simulink model "sdruqpskrx"  (R2025b)
settings: Solver=FixedStepDiscrete  StartTime=0.0  StopTime=inf  RelTol=1e-3
PreLoadFcn:
  | platform = sdruExampleFindRadio;
  | sdrqpskrx = sdruQPSKReceiverSLInit(platform, false, true);
  | clear platform
PostLoadFcn:
  | sdruExampleSetAvailableRadio;
InitFcn:
  | platform = get_param([gcs '/USRP Receiver'], 'Platform');
  | sdrqpskrx = sdruQPSKReceiverSLInit(platform, false, true);
  | switch platform
  |   case 'X300'
  |     set_param([gcs,'/USRP Receiver'], 'masterClkRateX300','200e6');
  |   case 'X310'
  |     set_param([gcs,'/USRP Receiver'], 'masterClkRateX310','200e6');
  |   case 'X410'
  |     set_param([gcs,'/USRP Receiver'], 'masterClkRateX410','250e6');
  |   case 'E320'
  |     set_param([gcs,'/USRP Receiver'], 'masterClkRateE320','50e6');
  |   case 'N300'
  |     set_param([gcs,'/USRP Receiver'], 'masterClkRateN300','125e6');
  |   case 'N310'
  |     set_param([gcs,'/USRP Receiver'], 'masterClkRateN310','125e6');
  |   case 'N320/N321'
  |      set_param([gcs,'/USRP Receiver'], 'masterClkRateN320','200e6');
  | end
  | clear platform
undefined symbols (not defined in the file): RX, TX
libraries: commrfcorlib x2, dspstat3 x2, commdigbbndpm3 x2, commsync2 x2, commrflib2 x1, dspsigops x1, simulink x1, commsequence2 x1, commsink2 x1, commutil2 x1, dspsrcs4 x1, commfilt2 x1
settings Model: FPTRunName=Active  SimulationMode=accelerator  Creator=The MathWorks, Inc.  LastModifiedBy=MiguelG
settings SolverCC: AlgebraicLoopSolver=TrustRegion  AutoInsertRateTranBlk=on  MaxZcPerStep=1.0
settings DataIOCC: LimitDataPoints=on  SaveFormat=Structure  SaveOutput=off  SignalLogging=off  DSMLogging=off  SaveTime=off  ReturnWorkspaceOutputs=off
settings OptimizationCC: DefaultParameterBehavior=Inlined  ReuseModelBlockBuffer=off  ExpressionDepthLimit=2147483647.0  LocalBlockOutputs=off  LifeSpan=inf  SimCompilerOptimization=on
settings DebuggingCC: AlgebraicLoopMsg=error  UnderspecifiedInitializationDetection=Classic  MergeDetectMultiDrivingBlocksExec=none  SolverPrmCheckMsg=warning  SingleTaskRateTransMsg=error  ParameterPrecisionLossMsg=none  FcnCallInpInsideContextMsg=warning  UnconnectedInputMsg=warning  UnconnectedOutputMsg=warning  UnconnectedLineMsg=warning  AllowSymbolicDim=off  StateNameClashWarn=warning  SFUnexpectedBacktrackingDiag=warning  SFNoUnconditionalDefaultTransitionDiag=warning  SFExecutionAtInitializationDiag=none  ArithmeticOperatorsInVariantConditions=warning
settings HardwareCC: ProdBitPerPointer=32.0  ProdBitPerSizeT=32.0  ProdBitPerPtrDiffT=32.0  ProdLargestAtomicFloat=None  ProdIntDivRoundTo=Undefined  ProdEndianess=Unspecified  ProdWordSize=32.0  ProdHWDeviceType=32-bit Generic  TargetBitPerPointer=64.0  TargetBitPerSizeT=64.0  TargetBitPerPtrDiffT=64.0  TargetLongLongMode=on  TargetIntDivRoundTo=Zero  TargetEndianess=LittleEndian  TargetWordSize=64.0  TargetHWDeviceType=Generic->MATLAB Host Computer  ProdEqTarget=off
settings ModelReferenceCC: EnableRefExpFcnMdlSchedulingChecks=on  PropagateSignalLabelsOutOfModel=off
settings SFSimCC: SimUseLocalCustomCode=off  CustomCodeUndefinedFunction=UseInterfaceOnly
settings RTWCC: RTWUseLocalCustomCode=off  GPUComputeCapability=3.5  DLArmComputeVersion=19.05
settings RTWCC: CustomSourceCode=|
  | #include <stdio.h>
  | #include <stdlib.h>
settings CodeAppCC: StateflowObjectComments=on
settings GRTTargetCC: TargetLangStandard=C89/C90 (ANSI)  CombineOutputUpdateFcns=off  GRTInterface=on
settings ConfigComp: CovMetricSettings=dw  CovSaveCumulativeToWorkspaceVar=on  CovSaveSingleToWorkspaceVar=on  CovExternalEMLEnable=off  CovSFcnEnable=off

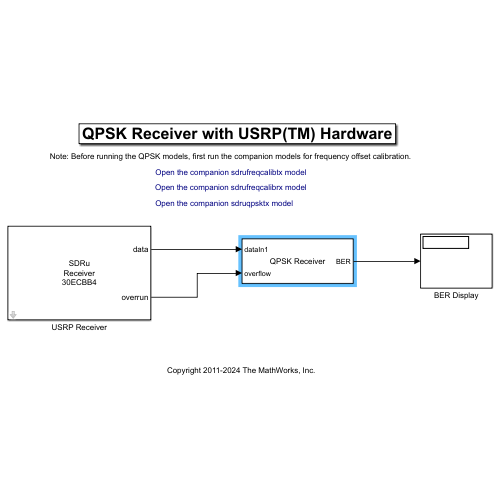
[thumbnail: Simulink's stored preview of the top-level diagram]
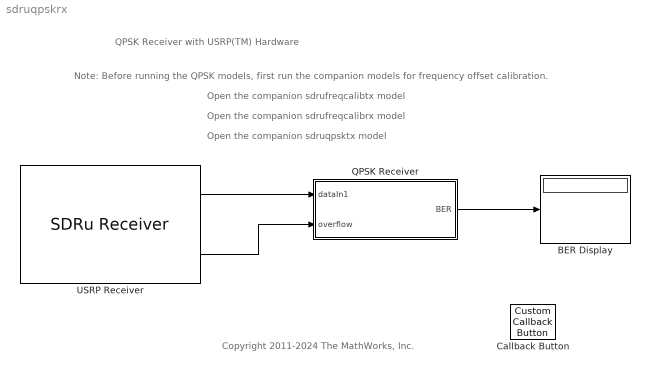
== system sdruqpskrx ==
  note: QPSK Receiver with USRP(TM) Hardware
  note: Open the companion sdruqpsktx model
  note: Note: Before running the QPSK models, first run the companion models for frequency offset calibration.
  note: Open the companion sdrufreqcalibrx model
  note: Open the companion sdrufreqcalibtx model
  note: Copyright 2011-2024 The MathWorks, Inc.
  BER Display : Display
  Callback Button : CustomCallbackButton  Configuration="{\"components\":[{\"name\":\"BackgroundImageComponent\",\"settings\":{\"image\":{\"size\":[0,0],\"src\":\"default\",\"srcOrientation\":\"Right\"},\"position\":[0,0,1,1]}},{\"name\":\"ButtonStateComponent\",\"settings\":{\"buttonType\":\"momentary\",\"clickFcn\":\"showExample('usrpradio\\/QPSKReceiverWithUSRPHardwareInSimulinkExample')\",\"onValue\":1,\"position\":[0,0,1,1],\"pressDelay\":\"500\",\"pressFcn\":\"\",\"repeatInterval\":\"0\",\"states\":[{\"horizontalAlignment\":\"center\",\"image\":{\"position\":[0,0,1,1],\"size\":[1,1],\"src\":\"default\",\"srcOrientation\":\"Right\"},\"label\":{\"color\":[0.01176470588,0.01176470588,0.01176470588,1],\"icon\":{\"size\":[0,0],\"src\":\"default\",\"srcOrientation\":\"Right\"},\"iconPlacement\":\"left\",\"opacity\":1,\"show\":true,\"text\":{\"content\":\"?\",\"font\":\"Helvetica\"}},\"labelOffset\":[0,0],\"verticalAlignment\":\"middle\"},{\"horizontalAlignment\":\"center\",\"image\":{\"position\":[0,0,1,1],\"size\":[1,1],\"src\":\"default\",\"srcOrientation\":\"Right\"},\"label\":{\"color\":[0.01176470588,0.01176470588,0.01176470588,1],\"icon\":{\"size\":[0,0],\"src\":\"default\",\"srcOrientation\":\"Right\"},\"iconPlacement\":\"left\",\"opacity\":1,\"show\":true,\"text\":{\"content\":\"?\",\"font\":\"Helvetica\"}},\"labelOffset\":[0,0],\"verticalAlignment\":\"middle\"},{\"horizontalAlignment\":\"center\",\"image\":{\"position\":[0,0,1,1],\"size\":[1,1],\"src\":\"default\",\"srcOrientation\":\"Right\"},\"label\":{\"color\":[0.01176470588,0.01176470588,0.01176470588,1],\"icon\":{\"size\":[0,0],\"src\":\"default\",\"srcOrientation\":\"Right\"},\"iconPlacement\":\"left\",\"opacity\":1,\"show\":true,\"text\":{\"content\":\"?\",\"font\":\"Helvetica\"}},\"labelOffset\":[0,0],\"verticalAlignment\":\"middle\"},{\"horizontalAlignment\":\"center\",\"image\":{\"position\":[0,0,1,1],\"size\":[1,1],\"src\":\"default\",\"srcOrientation\":\"Right\"},\"label\":{\"color\":[0.01176470588,0.01176470588,0.01176470588,1],\"icon\":{\"size\":[0,0],\"src\":\"default\",\"srcOrientation\":\"Right\"},\"iconPlacement\":\"left\",\"opacity\":1,\"show\":true,\"text\":{\"content\":\"?\",\"font\":\"Helvetica\"}},\"labelOffset\":[0,0],\"verticalAlignment\":\"middle\"}]}},{\"name\":\"ForegroundImageComponent\",\"settings\":{\"image\":{\"size\":[0,0],\"src\":\"default\",\"srcOrientation\":\"Right\"},\"isForeground\":1,\"position\":[0,0,1,1]}}],\"derived\":{\"blockParameters\":{\"AutoActivate\":true,\"ButtonText\":\"?\",\"ButtonType\":\"Momentary\",\"ClickFcn\":\"showExample('usrpradio\\/QPSKReceiverWithUSRPHardwareInSimulinkExample')\",\"OnValue\":1,\"PressDelay\":\"500\",\"PressFcn\":\"\",\"RepeatInterval\":\"0\",\"fixedAspectRatio\":\"off\"}},\"settings\":{\"BindingType\":\"standalone\",\"autoActivate\":true,\"backgroundColor\":[244,244,244,1],\"backgroundOffset\":0,\"backgroundOpacity\":1,\"fixedAspectRatio\":\"off\",\"foregroundColor\":[0.01176470588,0.01176470588,0.01176470588,1],\"migratedFromLegacy\":true,\"useBackgroundColor\":true,\"variant\":\"callback\",\"version\":\"R2025a\"},\"type\":\"Button\"}"  CustomBackgroundColor="{\"color\":[0.9568627451,0.9568627451,0.9568627451],\"show\":true}"
  QPSK Receiver : Subsystem
      mask Display: disp('QPSK Receiver')
  USRP Receiver : commsdrhw_v2/SDRu Receiver  rxtx=rx  initializeIPAddress=0  devMap=0  USRP2_IP=192.168.10.2  USRP_IP_X300=192.168.10.2  USRP_IP_X310=192.168.70.2  USRP_IP_N300=192.168.10.2  USRP_IP_N310=0.0.0.8  USRP_IP_N320=192.168.10.2  USRP_IP_E320=192.168.10.2  USRP_IP_X410=192.168.10.2  USRP_serialNumB200=30EA06C  USRP_serialNumB210=30ECBB4  platform=B210  prevPlatform=N200/N210/USRP2  lastIPAddressPopup=192.168.10.2  USRP_ID=30ECBB4  LastIPAddress=192.168.10.2  IsTwinRXDaughterboard=off  EnableTwinRXPhaseSync=off  losrc=0  ChannelMapping=1  rxAntennaPort=TX/RX  rxAntennaPortX410=RX1  centerFrequencySrc=Dialog  centerFrequency=sdrqpskrx.USRPCenterFrequency  loOffsetSrc=Dialog  loOffset=0  gainSrc=Dialog  gain=sdrqpskrx.USRPGain  PPSSource=Internal  clockSource=Internal  EnableGPSLock=off  EnsureSyncGPSTime=off  EnableTimeTrigger=off  triggerTime=5  enableMIMOCableSync=off  EnableRefLock=off  masterClkRateParam=20000000  masterClkRateB200=sdrqpskrx.MasterClockRate  masterClkRateB210=sdrqpskrx.MasterClockRate  masterClkRateX300=200e6  masterClkRateX310=200e6  masterClkRateN300=125e6  masterClkRateN310=125e6  masterClkRateN320=200e6  masterClkRateE320=30.72e6  masterClkRateX410=250e6  masterClkRate=100e6  masterClkRateTwinRX=200e6  decimInterpSrc=Dialog  decimInterpPort=512  lastDecimSource=Dialog  decimInterp=sdrqpskrx.USRPDecimationFactor  USRP2_IP_NUM=[51 48 69 67 66 66 52]  sampleRate=1000000  sampleTime=(20)/20000000  TransportDataType=int16  overrunUnderrunPort=on  dataLengthPort=off  EnableTimeStamps=off  outputDatatype=double  frameLength=sdrqpskrx.USRPFrameLength  HOST_DATA_PORT=0  HOST_CONTROL_PORT=0  USRP2_DATA_PORT=0  USRP2_CONTROL_PORT=0  bufferMode=Continuous streaming  EnableBurstMode=off  NumFramesInBurst=100
  wires:
  QPSK Receiver/1(BER) -> BER Display/1
  USRP Receiver/1 -> QPSK Receiver/1(dataIn1)
  USRP Receiver/2 -> QPSK Receiver/2(overflow)

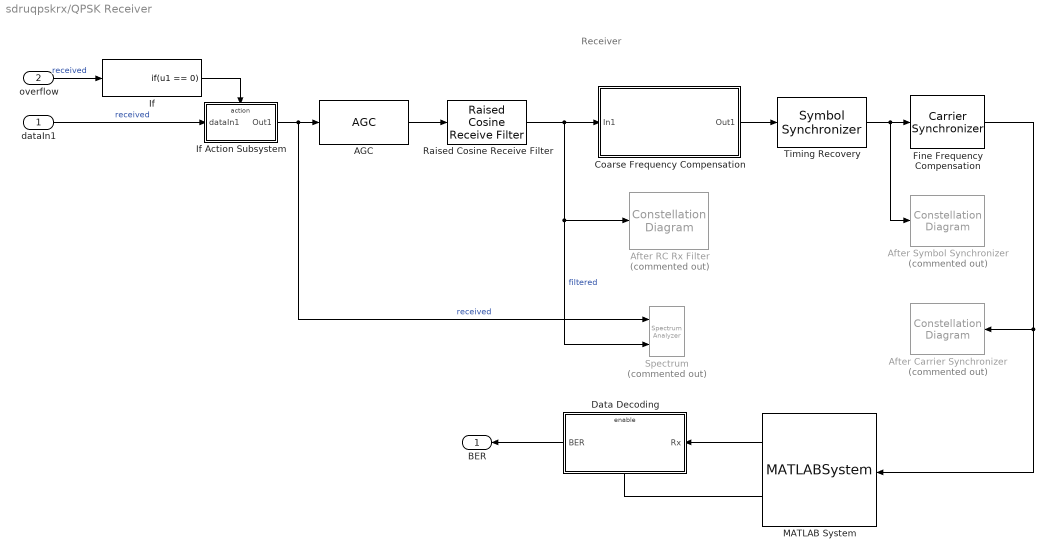
== system sdruqpskrx/QPSK Receiver ==
  note: Receiver
  dataIn1 : Inport
  overflow : Inport  Port=2
  AGC : commrfcorlib/AGC  LegacyMode=off  DetectorMethod=Rectifier  LoopMethod=Linear  UpdatePeriod=100  StepSize=0.1  AdaptationStepSize=0.01  DesiredOutputPower=sdrqpskrx.DesiredPower  AveragingLength=sdrqpskrx.AveragingLength  MaximumGain=30  MaxPowerGain=sdrqpskrx.MaxPowerGain  GainOutputPort=off  InputPowerOutputPort=off  SimulateUsing=Code generation
  After Carrier Synchronizer : ConstellationDiagram  Tag=ScatterPlot  Commented=on  SamplesPerSymbol=sdrqpskrx.Interpolation  SymbolsToDisplaySource=Property  SymbolsToDisplay=sdrqpskrx.FrameSize  ReferenceConstellation="{[1.4142+1.4142i          -1.4142+1.4142i          -1.4142-1.4142i           1.4142-1.4142i]}"  Title=After Carrier Synchronizer  XLimits=[-3 3]  YLimits=[-3 3]  AxesLimits=[-3 3]  EnableMeasurements=on  DefaultConfigurationName=comm.scopes.ConstellationDiagramBlockCfg
  After RC Rx Filter : ConstellationDiagram  Tag=ScatterPlot  Commented=on  SamplesPerSymbol=sdrqpskrx.Interpolation  SymbolsToDisplaySource=Property  SymbolsToDisplay=sdrqpskrx.FrameSize  ReferenceConstellation="{[1.4142+1.4142i          -1.4142+1.4142i          -1.4142-1.4142i           1.4142-1.4142i]}"  Title=After Raised Cosine Rx Filter  XLimits=[-3.1734 3.2134]  YLimits=[-3.1734 3.2134]  AxesLimits=[-3.1734 3.2134]  DefaultConfigurationName=comm.scopes.ConstellationDiagramBlockCfg
  After Symbol Synchronizer : ConstellationDiagram  Tag=ScatterPlot  Commented=on  SamplesPerSymbol=2  SymbolsToDisplaySource=Property  SymbolsToDisplay=sdrqpskrx.FrameSize  ReferenceConstellation="{[1.4142+1.4142i          -1.4142+1.4142i          -1.4142-1.4142i           1.4142-1.4142i]}"  Title=After Symbol Synchronizer  XLimits=[-3.0085 2.9872]  YLimits=[-3.0085 2.9872]  AxesLimits=[-3.0085 2.9872]  DefaultConfigurationName=comm.scopes.ConstellationDiagramBlockCfg
  Coarse Frequency Compensation : Subsystem
      mask Display: fprintf('Coarse Frequency\nCompensation')
  Data Decoding : Subsystem
      mask Display: disp('Data Decoding');
  Fine Frequency Compensation : commsync2/Carrier Synchronizer  Modulation=QPSK  ModulationPhaseOffset=Auto  CustomPhaseOffset=0  SamplesPerSymbol=sdrqpskrx.Interpolation/sdrqpskrx.Decimation  DampingFactor=1  NormalizedLoopBandwidth=0.01  EstimatedPhaseErrorOutputPort=off  SimulateUsing=Code generation
  If : If  IfExpression=u1 == 0  ShowElse=off
  If Action Subsystem : Subsystem  TreatAsAtomicUnit=on
  MATLAB System : MATLABSystem  System=FrameSynchronizer  Preamble=sqrt(2)/2 * (-1-1i) * (sdrqpskrx.BarkerCode)'  Threshold=0.9  OutputLength=sdrqpskrx.FrameSize  SimulateUsing=Code generation
      mask Type: FrameSynchronizer
  Raised Cosine Receive Filter : commfilt2/Raised Cosine Receive Filter  filtType=Square root  R=sdrqpskrx.RolloffFactor  filtSpan=sdrqpskrx.RaisedCosineFilterSpan  N=sdrqpskrx.Interpolation  downFactor=sdrqpskrx.Decimation  downOffset=0  filterGain=1  InputProcessing=Columns as channels (frame based)  RateOptions=Enforce single-rate processing  framing=Mute  checkCoeff=off  variableName=rcRxFilt  currentFiltSpan=10  D=5  inputOffset=0  sampMode=Mute  saveAsFlag=0  rateMode=Downsampling  checkGain=Normalized  launchFVT=on  roundingMode=Floor  overflowMode=off  coeffDataTypeStr=Inherit: Same word length as input  coeffMin=[]  coeffMax=[]  coeffLastDataTypeStr=Inherit: Same word length as input  accumDataTypeStr=Inherit: Same as product output  accumLastDataTypeStr=Inherit: Same as product output  outputDataTypeStr=Inherit: Same as accumulator  outputMin=[]  outputMax=[]  outputLastDataTypeStr=Inherit: Same as accumulator
  Spectrum : SpectrumAnalyzer  Commented=on  NumInputPorts=2  Method=Welch  SampleRate=100000  AxesScaling=Manual  RBWSource=Property  RBW=75  FFTLength=128  Span=100000  StartFrequency=-50000  StopFrequency=50000  AveragingMethod=Running  SpectralAverages=2  SpectrumUnits=dBW  Title=After Raised Cosine Rx Filter  YLabel=Power Spectrum  YLimits=[-137.6344738236879266 40]  ShowLegend=on  AllowFFTLengthLessThanSamplesPerUpdate=on
  Timing Recovery : commsync2/Symbol Synchronizer  Modulation=PAM/PSK/QAM  TimingErrorDetector=Gardner (non-data-aided)  SamplesPerSymbol=sdrqpskrx.Interpolation/sdrqpskrx.Decimation  DampingFactor=1  NormalizedLoopBandwidth=0.01  DetectorGain=sdrqpskrx.TimingErrorDetectorGain  TimingErrorOutputPort=off  SimulateUsing=Code generation
  BER : Outport  VectorParamsAs1DForOutWhenUnconnected=off
  wires:
  Raised Cosine Receive Filter/1 -> Coarse Frequency Compensation/1(In1), Spectrum/2, After RC Rx Filter/1  "filtered"
  Coarse Frequency Compensation/1(Out1) -> Timing Recovery/1
  Data Decoding/1(BER) -> BER/1
  AGC/1 -> Raised Cosine Receive Filter/1
  Fine Frequency Compensation/1 -> After Carrier Synchronizer/1, MATLAB System/1
  Timing Recovery/1 -> Fine Frequency Compensation/1, After Symbol Synchronizer/1
  If Action Subsystem/1(Out1) -> Spectrum/1, AGC/1  "received"
  overflow/1 -> If/1  "received"
  dataIn1/1 -> If Action Subsystem/1(dataIn1)  "received"
  If/1 -> If Action Subsystem/Action
  MATLAB System/1 -> Data Decoding/1(Rx)
  MATLAB System/2 -> Data Decoding/Enable

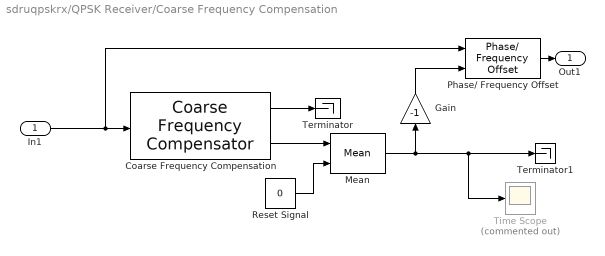
== system sdruqpskrx/QPSK Receiver/Coarse Frequency Compensation ==
  In1 : Inport
  Coarse Frequency Compensation : commrfcorlib/Coarse Frequency Compensator  Modulation=QPSK  Algorithm=Correlation-based  FrequencyResolution=25  MaximumFrequencyOffset=12.5e3  SamplesPerSymbol=4  EstimatedFreqOffsetPort=on  SimulateUsing=Code generation
  Gain : Gain  Gain=-1
  Mean : dspstat3/Mean  run=on  InputProcessing=Columns as channels (frame based)  reset_popup=Either edge  directionMode=Each column  dimension=1  roiEnable=off  roiType=Rectangles  roiPortion=Entire ROI  roiOutput=Individual statistics for each ROI  roiFlag=off  roundingMode=Floor  overflowMode=off  outputDataTypeStr=Inherit: Same as accumulator  outputMin=[]  outputMax=[]  outputLastDataTypeStr=Inherit: Same as accumulator
  Phase/ Frequency Offset : commrflib2/Phase// Frequency Offset  phaseOffset=0  freqPort=on  freqOffset=0
  Reset Signal : Constant  Value=0
  Terminator : Terminator
  Terminator1 : Terminator
  Time Scope : Scope  Commented=on
      settings: TimeUnits=Metric (based on Time Span)  YLabel=Amplitude
  Out1 : Outport  VectorParamsAs1DForOutWhenUnconnected=off
  wires:
  In1/1 -> Phase/ Frequency Offset/1, Coarse Frequency Compensation/1
  Phase/ Frequency Offset/1 -> Out1/1
  Mean/1 -> Time Scope/1, Terminator1/1, Gain/1
  Coarse Frequency Compensation/2 -> Mean/1
  Coarse Frequency Compensation/1 -> Terminator/1
  Gain/1 -> Phase/ Frequency Offset/2
  Reset Signal/1 -> Mean/2

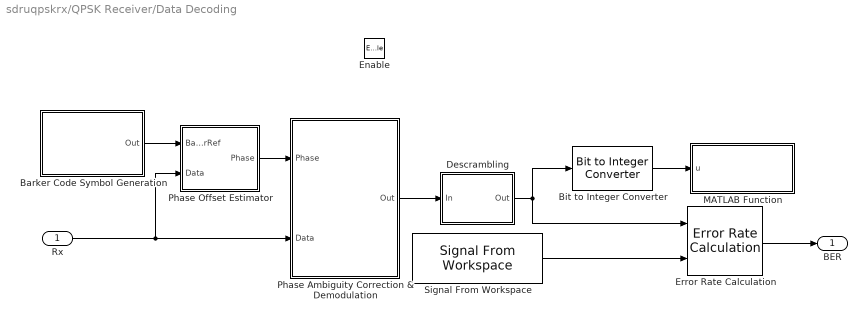
== system sdruqpskrx/QPSK Receiver/Data Decoding ==
  Rx : Inport
  Enable : EnablePort
  "Barker Code Symbol Generation " : Subsystem
      mask Display: disp('Barker Code\nSymbol Generation')
  Bit to Integer Converter : simulink/Logic and Bit Operations/Bit to Integer Converter  nbits=7  bitOrder=MSB first  signedOutputValues=Unsigned  outDtype=Inherit via internal rule  outDtypeSigned=Inherit via internal rule
  Descrambling : Subsystem
      mask Display: disp('Descrambling');
  Error Rate Calculation : commsink2/Error Rate Calculation  N=0  st_delay=0  cp_mode=Select samples from mask  subframe=sdrqpskrx.BerMask  PMode=Port  WsName=ErrorVec  RsMode2=off  stop=off  numErr=100  maxBits=1e6
  MATLAB Function : MATLAB Function  TreatAsAtomicUnit=on
  Phase Ambiguity Correction & Demodulation : Subsystem
      mask Display: disp('Phase Ambiguity\nCorrection\n& Demodulation');
  Phase Offset Estimator : Subsystem
  Signal From Workspace : dspsrcs4/Signal From Workspace  X=sdrqpskrx.MessageBits  Ts=1/sdrqpskrx.PayloadLength*sdrqpskrx.FrameTime  nsamps=sdrqpskrx.MessageLength * 7 * sdrqpskrx.NumberOfMessage  OutputAfterFinalValue=Cyclic repetition  ignoreOrWarnInputAndFrameLengths=off  OutputFrames=off
  BER : Outport  VectorParamsAs1DForOutWhenUnconnected=off
  wires:
  "Barker Code Symbol Generation "/1(Out) -> Phase Offset Estimator/1(BarkerRef)
  Phase Offset Estimator/1(Phase) -> Phase Ambiguity Correction & Demodulation/1(Phase)
  Rx/1 -> Phase Offset Estimator/2(Data), Phase Ambiguity Correction & Demodulation/2(Data)
  Descrambling/1(Out) -> Error Rate Calculation/1, Bit to Integer Converter/1
  Error Rate Calculation/1 -> BER/1
  Phase Ambiguity Correction & Demodulation/1(Out) -> Descrambling/1(In)
  Signal From Workspace/1 -> Error Rate Calculation/2
  Bit to Integer Converter/1 -> MATLAB Function/1(u)

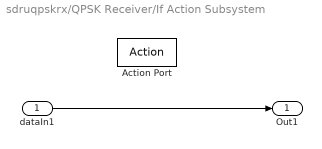
== system sdruqpskrx/QPSK Receiver/If Action Subsystem ==
  dataIn1 : Inport
  Action Port : ActionPort  ActionPortLabel=if(u1 == 0)
  Out1 : Outport
  wires:
  dataIn1/1 -> Out1/1

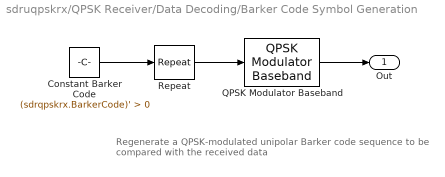
== system sdruqpskrx/QPSK Receiver/Data Decoding/Barker Code Symbol Generation  ==
  note: Regenerate a QPSK-modulated unipolar Barker code sequence
      | to be compared with the received data
  Constant Barker Code : Constant  Value=(sdrqpskrx.BarkerCode)' > 0  VectorParams1D=off  OutDataTypeStr=double
  QPSK Modulator Baseband : commdigbbndpm3/QPSK Modulator Baseband  InType=Bit  Enc=Gray  Ph=pi/4  outDtype=double  outWordLen=16  outUDDataType=sfix(16)  outFracLenMode=Best precision  outFracLen=15  outDataTypeStr=double  outLastDataTypeStr=double
  Repeat : dspsigops/Repeat  FactorSource=Dialog parameter  N=2  Nmax=16  InputProcessing=Columns as channels (frame based)  RateOptions=Enforce single-rate processing  ic=0  mode=Unused parameter value
  Out : Outport  VectorParamsAs1DForOutWhenUnconnected=off
  wires:
  Constant Barker Code/1 -> Repeat/1
  Repeat/1 -> QPSK Modulator Baseband/1
  QPSK Modulator Baseband/1 -> Out/1

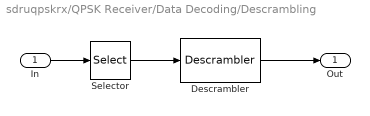
== system sdruqpskrx/QPSK Receiver/Data Decoding/Descrambling ==
  In : Inport
  Descrambler : commsequence2/Descrambler  M=2  poly=[1 1 1 0 1]  iniStaSource=Dialog Parameter  ini_sta=[0 0 0 0]  resetViaPort=off
  Selector : Selector  IndexOptions=Index vector (dialog)  Indices=[sdrqpskrx.HeaderLength+(1 : sdrqpskrx.PayloadLength)]  OutputSizes=1
  Out : Outport  VectorParamsAs1DForOutWhenUnconnected=off
  wires:
  In/1 -> Selector/1
  Selector/1 -> Descrambler/1
  Descrambler/1 -> Out/1

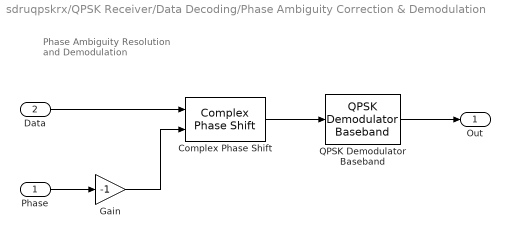
== system sdruqpskrx/QPSK Receiver/Data Decoding/Phase Ambiguity Correction & Demodulation ==
  note: Phase Ambiguity Resolution
      | and Demodulation
  Phase : Inport
  Data : Inport  Port=2
  Complex Phase Shift : commutil2/Complex Phase Shift
  Gain : Gain  Gain=-1  OutDataTypeStr=Inherit: Same as input
  QPSK Demodulator Baseband : commdigbbndpm3/QPSK Demodulator Baseband  OutType=Bit  DecType=Hard decision  VarSource=Dialog  Variance=1  Dec=Gray  Ph=pi/4  outDtype1=Inherit via internal rule  outDtype2=Inherit via internal rule  derotateFactorWordLen=16  derotateFactorDataTypeStr=Inherit: Same word length as input  derotateFactorLastDataTypeStr=Inherit: Same word length as input
  Out : Outport  VectorParamsAs1DForOutWhenUnconnected=off
  wires:
  Phase/1 -> Gain/1
  Data/1 -> Complex Phase Shift/1
  Complex Phase Shift/1 -> QPSK Demodulator Baseband/1
  QPSK Demodulator Baseband/1 -> Out/1
  Gain/1 -> Complex Phase Shift/2

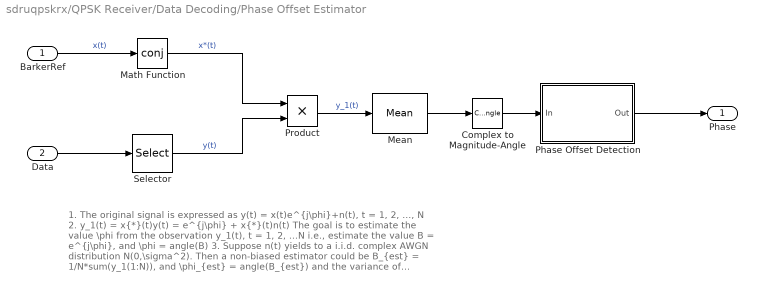
== system sdruqpskrx/QPSK Receiver/Data Decoding/Phase Offset Estimator ==
  note: 1. The original signal is expressed as y(t) = x(t)e^{j\phi}+n(t), t = 1, 2, ..., N
      | 2. y_1(t) = x{*}(t)y(t) = e^{j\phi} + x{*}(t)n(t)
      | The goal is to estimate the value \phi from the observation y_1(t), t = 1, 2, ...N
      | i.e., estimate the value B = e^{j\phi}, and \phi = angle(B)
      | 3. Suppose n(t) yields to a i.i.d. complex AWGN distribution N(0,\sigma^2).
      | Then a non-biased estimator could be
      | B_{est} = 1/N*sum(y_1(1:N)), and \phi_{est} = angle(B_{est})
      | and the variance of B_{est} is \sigma^2/N
  BarkerRef : Inport
  Data : Inport  Port=2
  Complex to Magnitude-Angle : ComplexToMagnitudeAngle  Output=Angle
  Math Function : Math  Operator=conj  SignedPower=on
  Mean : dspstat3/Mean  run=off  InputProcessing=Columns as channels (frame based)  reset_popup=None  directionMode=Each column  dimension=1  roiEnable=off  roiType=Rectangles  roiPortion=Entire ROI  roiOutput=Individual statistics for each ROI  roiFlag=off  roundingMode=Floor  overflowMode=off  outputDataTypeStr=Inherit: Same as accumulator  outputMin=[]  outputMax=[]  outputLastDataTypeStr=Inherit: Same as accumulator
  Phase Offset Detection : MATLAB Function  TreatAsAtomicUnit=on
  Product : Product  RndMeth=Zero
  Selector : Selector  IndexOptions=Index vector (dialog)  Indices=[1:sdrqpskrx.BarkerLength]  OutputSizes=1
  Phase : Outport  VectorParamsAs1DForOutWhenUnconnected=off
  wires:
  Data/1 -> Selector/1
  BarkerRef/1 -> Math Function/1  "x(t)"
  Selector/1 -> Product/2  "y(t)"
  Math Function/1 -> Product/1  "x*(t)"
  Product/1 -> Mean/1  "y_1(t)"
  Mean/1 -> Complex to Magnitude-Angle/1
  Complex to Magnitude-Angle/1 -> Phase Offset Detection/1(In)
  Phase Offset Detection/1(Out) -> Phase/1

== matlab function sdruqpskrx/QPSK Receiver/Data Decoding/Phase Offset Estimator/Phase Offset Detection ==
  data: In input; Out output
function Out = phasedecision(In)
% Map the estimated phase to one of -pi, -pi/2, 0, pi/2,  
%#codegen
Out = round(In.*2./pi)./2.*pi;
% The above processing is equivalent to the following processing using
% if/else statements
%
% if In<pi/4 && In>-pi/4
%     Out = 0;
% elseif In>=pi/4 && In<pi*3/4
%     Out = pi/2;
% elseif In>=pi*3/4 || In<=-pi*3/4
%     Out = -pi;
% else
%     Out = -pi/2;
% end

== matlab function sdruqpskrx/QPSK Receiver/Data Decoding/MATLAB Function ==
  data: u input
function IntegerToASCII(u)
    fprintf('%s', char(u'));
end
